simulink model "nn_plus"  (R2018b)
settings: Solver=VariableStepAuto  StartTime=0.0  StopTime=10.0  RelTol=1e-3
libraries: neural x265
(part 2 of 2)

== system nn_plus/LSTM SHA2/LSTMM Cell (with XOR|AND|SUM encapsulation)1/LSTM | XOR |AND (NN)/SUM NN/LSTM Cell [t] ==
  C[t-1] : Inport
  h[t-1] : Inport  Port=2
  X1 : Inport  Port=3
  X2 : Inport  Port=4
  Product : Product
  Product1 : Product
  Sum : Sum  Inputs=|++
  Sum1 : Sum  Inputs=|++
  Vector Concatenate : Concatenate  NumInputs=3
  logsig : neural/Transfer Functions/logsig
  logsig1 : neural/Transfer Functions/logsig
  logsig2 : neural/Transfer Functions/logsig
  tansig3 : neural/Transfer Functions/tansig
  tansig4 : neural/Transfer Functions/tansig
  C[t] : Outport
  h[t] : Outport  Port=2
  wires:
  h[t-1]/1 -> Vector Concatenate/1
  X1/1 -> Vector Concatenate/2
  X2/1 -> Vector Concatenate/3
  Vector Concatenate/1 -> tansig3/1, logsig2/1, logsig1/1, logsig/1
  C[t-1]/1 -> Sum/1
  logsig/1 -> Sum/2
  Sum/1 -> Sum1/1
  tansig3/1 -> Product/2
  logsig1/1 -> Product/1
  Product/1 -> Sum1/2
  logsig2/1 -> Product1/2
  Sum1/1 -> C[t]/1, tansig4/1
  tansig4/1 -> Product1/1
  Product1/1 -> h[t]/1

== system nn_plus/LSTM SHA2/LSTMM Cell (with XOR|AND|SUM encapsulation)1/LSTM | XOR |AND (NN)/SUM NN/LSTM Cell[t=1] ==
  note: LSTM Cell L1 (Block-Scheme)
  C[t-1] : Inport
  h[t-1] : Inport  Port=2
  X1 : Inport  Port=3
  X2 : Inport  Port=4
  Product : Product
  Product1 : Product
  Sum : Sum  Inputs=|++
  Sum1 : Sum  Inputs=|++
  Vector Concatenate : Concatenate  NumInputs=3
  logsig : neural/Transfer Functions/logsig
  logsig1 : neural/Transfer Functions/logsig
  logsig2 : neural/Transfer Functions/logsig
  tansig3 : neural/Transfer Functions/tansig
  tansig4 : neural/Transfer Functions/tansig
  C[t] : Outport
  h[t] : Outport  Port=2
  wires:
  h[t-1]/1 -> Vector Concatenate/1
  X1/1 -> Vector Concatenate/2
  X2/1 -> Vector Concatenate/3
  Vector Concatenate/1 -> logsig/1, logsig2/1, tansig3/1, logsig1/1
  C[t-1]/1 -> Sum/1
  logsig/1 -> Sum/2
  Sum/1 -> Sum1/1
  tansig3/1 -> Product/2
  logsig1/1 -> Product/1
  Product/1 -> Sum1/2
  logsig2/1 -> Product1/2
  Sum1/1 -> C[t]/1, tansig4/1
  tansig4/1 -> Product1/1
  Product1/1 -> h[t]/1

== system nn_plus/LSTM SHA2/LSTMM Cell (with XOR|AND|SUM encapsulation)1/LSTM | XOR |AND (NN)/SUM NN/LSTM Cell[t=2] ==
  C[t-1] : Inport
  h[t-1] : Inport  Port=2
  X1 : Inport  Port=3
  X2 : Inport  Port=4
  Product : Product
  Product1 : Product
  Sum : Sum  Inputs=|++
  Sum1 : Sum  Inputs=|++
  Vector Concatenate : Concatenate  NumInputs=3
  logsig : neural/Transfer Functions/logsig
  logsig1 : neural/Transfer Functions/logsig
  logsig2 : neural/Transfer Functions/logsig
  tansig3 : neural/Transfer Functions/tansig
  tansig4 : neural/Transfer Functions/tansig
  C[t] : Outport
  h[t] : Outport  Port=2
  wires:
  h[t-1]/1 -> Vector Concatenate/1
  X1/1 -> Vector Concatenate/2
  X2/1 -> Vector Concatenate/3
  Vector Concatenate/1 -> tansig3/1, logsig2/1, logsig1/1, logsig/1
  C[t-1]/1 -> Sum/1
  logsig/1 -> Sum/2
  Sum/1 -> Sum1/1
  tansig3/1 -> Product/2
  logsig1/1 -> Product/1
  Product/1 -> Sum1/2
  logsig2/1 -> Product1/2
  Sum1/1 -> C[t]/1, tansig4/1
  tansig4/1 -> Product1/1
  Product1/1 -> h[t]/1

== system nn_plus/LSTM SHA2/LSTMM Cell (with XOR|AND|SUM encapsulation)2/LSTM | XOR |AND (NN)/SUM NN/LSTM Cell [t=31] ==
  C[t-1] : Inport
  h[t-1] : Inport  Port=2
  X1 : Inport  Port=3
  X2 : Inport  Port=4
  Product : Product
  Product1 : Product
  Sum : Sum  Inputs=|++
  Sum1 : Sum  Inputs=|++
  Vector Concatenate : Concatenate  NumInputs=3
  logsig : neural/Transfer Functions/logsig
  logsig1 : neural/Transfer Functions/logsig
  logsig2 : neural/Transfer Functions/logsig
  tansig3 : neural/Transfer Functions/tansig
  tansig4 : neural/Transfer Functions/tansig
  C[t] : Outport
  h[t] : Outport  Port=2
  wires:
  h[t-1]/1 -> Vector Concatenate/1
  X1/1 -> Vector Concatenate/2
  X2/1 -> Vector Concatenate/3
  Vector Concatenate/1 -> tansig3/1, logsig2/1, logsig1/1, logsig/1
  C[t-1]/1 -> Sum/1
  logsig/1 -> Sum/2
  Sum/1 -> Sum1/1
  tansig3/1 -> Product/2
  logsig1/1 -> Product/1
  Product/1 -> Sum1/2
  logsig2/1 -> Product1/2
  Sum1/1 -> C[t]/1, tansig4/1
  tansig4/1 -> Product1/1
  Product1/1 -> h[t]/1

== system nn_plus/LSTM SHA2/LSTMM Cell (with XOR|AND|SUM encapsulation)2/LSTM | XOR |AND (NN)/SUM NN/LSTM Cell [t] ==
  C[t-1] : Inport
  h[t-1] : Inport  Port=2
  X1 : Inport  Port=3
  X2 : Inport  Port=4
  Product : Product
  Product1 : Product
  Sum : Sum  Inputs=|++
  Sum1 : Sum  Inputs=|++
  Vector Concatenate : Concatenate  NumInputs=3
  logsig : neural/Transfer Functions/logsig
  logsig1 : neural/Transfer Functions/logsig
  logsig2 : neural/Transfer Functions/logsig
  tansig3 : neural/Transfer Functions/tansig
  tansig4 : neural/Transfer Functions/tansig
  C[t] : Outport
  h[t] : Outport  Port=2
  wires:
  h[t-1]/1 -> Vector Concatenate/1
  X1/1 -> Vector Concatenate/2
  X2/1 -> Vector Concatenate/3
  Vector Concatenate/1 -> tansig3/1, logsig2/1, logsig1/1, logsig/1
  C[t-1]/1 -> Sum/1
  logsig/1 -> Sum/2
  Sum/1 -> Sum1/1
  tansig3/1 -> Product/2
  logsig1/1 -> Product/1
  Product/1 -> Sum1/2
  logsig2/1 -> Product1/2
  Sum1/1 -> C[t]/1, tansig4/1
  tansig4/1 -> Product1/1
  Product1/1 -> h[t]/1

== system nn_plus/LSTM SHA2/LSTMM Cell (with XOR|AND|SUM encapsulation)2/LSTM | XOR |AND (NN)/SUM NN/LSTM Cell[t=1] ==
  note: LSTM Cell L1 (Block-Scheme)
  C[t-1] : Inport
  h[t-1] : Inport  Port=2
  X1 : Inport  Port=3
  X2 : Inport  Port=4
  Product : Product
  Product1 : Product
  Sum : Sum  Inputs=|++
  Sum1 : Sum  Inputs=|++
  Vector Concatenate : Concatenate  NumInputs=3
  logsig : neural/Transfer Functions/logsig
  logsig1 : neural/Transfer Functions/logsig
  logsig2 : neural/Transfer Functions/logsig
  tansig3 : neural/Transfer Functions/tansig
  tansig4 : neural/Transfer Functions/tansig
  C[t] : Outport
  h[t] : Outport  Port=2
  wires:
  h[t-1]/1 -> Vector Concatenate/1
  X1/1 -> Vector Concatenate/2
  X2/1 -> Vector Concatenate/3
  Vector Concatenate/1 -> logsig/1, logsig2/1, tansig3/1, logsig1/1
  C[t-1]/1 -> Sum/1
  logsig/1 -> Sum/2
  Sum/1 -> Sum1/1
  tansig3/1 -> Product/2
  logsig1/1 -> Product/1
  Product/1 -> Sum1/2
  logsig2/1 -> Product1/2
  Sum1/1 -> C[t]/1, tansig4/1
  tansig4/1 -> Product1/1
  Product1/1 -> h[t]/1

== system nn_plus/LSTM SHA2/LSTMM Cell (with XOR|AND|SUM encapsulation)2/LSTM | XOR |AND (NN)/SUM NN/LSTM Cell[t=2] ==
  C[t-1] : Inport
  h[t-1] : Inport  Port=2
  X1 : Inport  Port=3
  X2 : Inport  Port=4
  Product : Product
  Product1 : Product
  Sum : Sum  Inputs=|++
  Sum1 : Sum  Inputs=|++
  Vector Concatenate : Concatenate  NumInputs=3
  logsig : neural/Transfer Functions/logsig
  logsig1 : neural/Transfer Functions/logsig
  logsig2 : neural/Transfer Functions/logsig
  tansig3 : neural/Transfer Functions/tansig
  tansig4 : neural/Transfer Functions/tansig
  C[t] : Outport
  h[t] : Outport  Port=2
  wires:
  h[t-1]/1 -> Vector Concatenate/1
  X1/1 -> Vector Concatenate/2
  X2/1 -> Vector Concatenate/3
  Vector Concatenate/1 -> tansig3/1, logsig2/1, logsig1/1, logsig/1
  C[t-1]/1 -> Sum/1
  logsig/1 -> Sum/2
  Sum/1 -> Sum1/1
  tansig3/1 -> Product/2
  logsig1/1 -> Product/1
  Product/1 -> Sum1/2
  logsig2/1 -> Product1/2
  Sum1/1 -> C[t]/1, tansig4/1
  tansig4/1 -> Product1/1
  Product1/1 -> h[t]/1

== system nn_plus/LSTM SHA2/LSTMM Cell (with XOR|AND|SUM encapsulation)3/LSTM | XOR |AND (NN)/SUM NN/LSTM Cell [t=31] ==
  C[t-1] : Inport
  h[t-1] : Inport  Port=2
  X1 : Inport  Port=3
  X2 : Inport  Port=4
  Product : Product
  Product1 : Product
  Sum : Sum  Inputs=|++
  Sum1 : Sum  Inputs=|++
  Vector Concatenate : Concatenate  NumInputs=3
  logsig : neural/Transfer Functions/logsig
  logsig1 : neural/Transfer Functions/logsig
  logsig2 : neural/Transfer Functions/logsig
  tansig3 : neural/Transfer Functions/tansig
  tansig4 : neural/Transfer Functions/tansig
  C[t] : Outport
  h[t] : Outport  Port=2
  wires:
  h[t-1]/1 -> Vector Concatenate/1
  X1/1 -> Vector Concatenate/2
  X2/1 -> Vector Concatenate/3
  Vector Concatenate/1 -> tansig3/1, logsig2/1, logsig1/1, logsig/1
  C[t-1]/1 -> Sum/1
  logsig/1 -> Sum/2
  Sum/1 -> Sum1/1
  tansig3/1 -> Product/2
  logsig1/1 -> Product/1
  Product/1 -> Sum1/2
  logsig2/1 -> Product1/2
  Sum1/1 -> C[t]/1, tansig4/1
  tansig4/1 -> Product1/1
  Product1/1 -> h[t]/1

== system nn_plus/LSTM SHA2/LSTMM Cell (with XOR|AND|SUM encapsulation)3/LSTM | XOR |AND (NN)/SUM NN/LSTM Cell [t] ==
  C[t-1] : Inport
  h[t-1] : Inport  Port=2
  X1 : Inport  Port=3
  X2 : Inport  Port=4
  Product : Product
  Product1 : Product
  Sum : Sum  Inputs=|++
  Sum1 : Sum  Inputs=|++
  Vector Concatenate : Concatenate  NumInputs=3
  logsig : neural/Transfer Functions/logsig
  logsig1 : neural/Transfer Functions/logsig
  logsig2 : neural/Transfer Functions/logsig
  tansig3 : neural/Transfer Functions/tansig
  tansig4 : neural/Transfer Functions/tansig
  C[t] : Outport
  h[t] : Outport  Port=2
  wires:
  h[t-1]/1 -> Vector Concatenate/1
  X1/1 -> Vector Concatenate/2
  X2/1 -> Vector Concatenate/3
  Vector Concatenate/1 -> tansig3/1, logsig2/1, logsig1/1, logsig/1
  C[t-1]/1 -> Sum/1
  logsig/1 -> Sum/2
  Sum/1 -> Sum1/1
  tansig3/1 -> Product/2
  logsig1/1 -> Product/1
  Product/1 -> Sum1/2
  logsig2/1 -> Product1/2
  Sum1/1 -> C[t]/1, tansig4/1
  tansig4/1 -> Product1/1
  Product1/1 -> h[t]/1

== system nn_plus/LSTM SHA2/LSTMM Cell (with XOR|AND|SUM encapsulation)3/LSTM | XOR |AND (NN)/SUM NN/LSTM Cell[t=1] ==
  note: LSTM Cell L1 (Block-Scheme)
  C[t-1] : Inport
  h[t-1] : Inport  Port=2
  X1 : Inport  Port=3
  X2 : Inport  Port=4
  Product : Product
  Product1 : Product
  Sum : Sum  Inputs=|++
  Sum1 : Sum  Inputs=|++
  Vector Concatenate : Concatenate  NumInputs=3
  logsig : neural/Transfer Functions/logsig
  logsig1 : neural/Transfer Functions/logsig
  logsig2 : neural/Transfer Functions/logsig
  tansig3 : neural/Transfer Functions/tansig
  tansig4 : neural/Transfer Functions/tansig
  C[t] : Outport
  h[t] : Outport  Port=2
  wires:
  h[t-1]/1 -> Vector Concatenate/1
  X1/1 -> Vector Concatenate/2
  X2/1 -> Vector Concatenate/3
  Vector Concatenate/1 -> logsig/1, logsig2/1, tansig3/1, logsig1/1
  C[t-1]/1 -> Sum/1
  logsig/1 -> Sum/2
  Sum/1 -> Sum1/1
  tansig3/1 -> Product/2
  logsig1/1 -> Product/1
  Product/1 -> Sum1/2
  logsig2/1 -> Product1/2
  Sum1/1 -> C[t]/1, tansig4/1
  tansig4/1 -> Product1/1
  Product1/1 -> h[t]/1

== system nn_plus/LSTM SHA2/LSTMM Cell (with XOR|AND|SUM encapsulation)3/LSTM | XOR |AND (NN)/SUM NN/LSTM Cell[t=2] ==
  C[t-1] : Inport
  h[t-1] : Inport  Port=2
  X1 : Inport  Port=3
  X2 : Inport  Port=4
  Product : Product
  Product1 : Product
  Sum : Sum  Inputs=|++
  Sum1 : Sum  Inputs=|++
  Vector Concatenate : Concatenate  NumInputs=3
  logsig : neural/Transfer Functions/logsig
  logsig1 : neural/Transfer Functions/logsig
  logsig2 : neural/Transfer Functions/logsig
  tansig3 : neural/Transfer Functions/tansig
  tansig4 : neural/Transfer Functions/tansig
  C[t] : Outport
  h[t] : Outport  Port=2
  wires:
  h[t-1]/1 -> Vector Concatenate/1
  X1/1 -> Vector Concatenate/2
  X2/1 -> Vector Concatenate/3
  Vector Concatenate/1 -> tansig3/1, logsig2/1, logsig1/1, logsig/1
  C[t-1]/1 -> Sum/1
  logsig/1 -> Sum/2
  Sum/1 -> Sum1/1
  tansig3/1 -> Product/2
  logsig1/1 -> Product/1
  Product/1 -> Sum1/2
  logsig2/1 -> Product1/2
  Sum1/1 -> C[t]/1, tansig4/1
  tansig4/1 -> Product1/1
  Product1/1 -> h[t]/1

== system nn_plus/LSTM SHA2/LSTMM Cell (with XOR|AND|SUM encapsulation)4/LSTM | XOR |AND (NN)/SUM NN/LSTM Cell [t=31] ==
  C[t-1] : Inport
  h[t-1] : Inport  Port=2
  X1 : Inport  Port=3
  X2 : Inport  Port=4
  Product : Product
  Product1 : Product
  Sum : Sum  Inputs=|++
  Sum1 : Sum  Inputs=|++
  Vector Concatenate : Concatenate  NumInputs=3
  logsig : neural/Transfer Functions/logsig
  logsig1 : neural/Transfer Functions/logsig
  logsig2 : neural/Transfer Functions/logsig
  tansig3 : neural/Transfer Functions/tansig
  tansig4 : neural/Transfer Functions/tansig
  C[t] : Outport
  h[t] : Outport  Port=2
  wires:
  h[t-1]/1 -> Vector Concatenate/1
  X1/1 -> Vector Concatenate/2
  X2/1 -> Vector Concatenate/3
  Vector Concatenate/1 -> tansig3/1, logsig2/1, logsig1/1, logsig/1
  C[t-1]/1 -> Sum/1
  logsig/1 -> Sum/2
  Sum/1 -> Sum1/1
  tansig3/1 -> Product/2
  logsig1/1 -> Product/1
  Product/1 -> Sum1/2
  logsig2/1 -> Product1/2
  Sum1/1 -> C[t]/1, tansig4/1
  tansig4/1 -> Product1/1
  Product1/1 -> h[t]/1

== system nn_plus/LSTM SHA2/LSTMM Cell (with XOR|AND|SUM encapsulation)4/LSTM | XOR |AND (NN)/SUM NN/LSTM Cell [t] ==
  C[t-1] : Inport
  h[t-1] : Inport  Port=2
  X1 : Inport  Port=3
  X2 : Inport  Port=4
  Product : Product
  Product1 : Product
  Sum : Sum  Inputs=|++
  Sum1 : Sum  Inputs=|++
  Vector Concatenate : Concatenate  NumInputs=3
  logsig : neural/Transfer Functions/logsig
  logsig1 : neural/Transfer Functions/logsig
  logsig2 : neural/Transfer Functions/logsig
  tansig3 : neural/Transfer Functions/tansig
  tansig4 : neural/Transfer Functions/tansig
  C[t] : Outport
  h[t] : Outport  Port=2
  wires:
  h[t-1]/1 -> Vector Concatenate/1
  X1/1 -> Vector Concatenate/2
  X2/1 -> Vector Concatenate/3
  Vector Concatenate/1 -> tansig3/1, logsig2/1, logsig1/1, logsig/1
  C[t-1]/1 -> Sum/1
  logsig/1 -> Sum/2
  Sum/1 -> Sum1/1
  tansig3/1 -> Product/2
  logsig1/1 -> Product/1
  Product/1 -> Sum1/2
  logsig2/1 -> Product1/2
  Sum1/1 -> C[t]/1, tansig4/1
  tansig4/1 -> Product1/1
  Product1/1 -> h[t]/1

== system nn_plus/LSTM SHA2/LSTMM Cell (with XOR|AND|SUM encapsulation)4/LSTM | XOR |AND (NN)/SUM NN/LSTM Cell[t=1] ==
  note: LSTM Cell L1 (Block-Scheme)
  C[t-1] : Inport
  h[t-1] : Inport  Port=2
  X1 : Inport  Port=3
  X2 : Inport  Port=4
  Product : Product
  Product1 : Product
  Sum : Sum  Inputs=|++
  Sum1 : Sum  Inputs=|++
  Vector Concatenate : Concatenate  NumInputs=3
  logsig : neural/Transfer Functions/logsig
  logsig1 : neural/Transfer Functions/logsig
  logsig2 : neural/Transfer Functions/logsig
  tansig3 : neural/Transfer Functions/tansig
  tansig4 : neural/Transfer Functions/tansig
  C[t] : Outport
  h[t] : Outport  Port=2
  wires:
  h[t-1]/1 -> Vector Concatenate/1
  X1/1 -> Vector Concatenate/2
  X2/1 -> Vector Concatenate/3
  Vector Concatenate/1 -> logsig/1, logsig2/1, tansig3/1, logsig1/1
  C[t-1]/1 -> Sum/1
  logsig/1 -> Sum/2
  Sum/1 -> Sum1/1
  tansig3/1 -> Product/2
  logsig1/1 -> Product/1
  Product/1 -> Sum1/2
  logsig2/1 -> Product1/2
  Sum1/1 -> C[t]/1, tansig4/1
  tansig4/1 -> Product1/1
  Product1/1 -> h[t]/1

== system nn_plus/LSTM SHA2/LSTMM Cell (with XOR|AND|SUM encapsulation)4/LSTM | XOR |AND (NN)/SUM NN/LSTM Cell[t=2] ==
  C[t-1] : Inport
  h[t-1] : Inport  Port=2
  X1 : Inport  Port=3
  X2 : Inport  Port=4
  Product : Product
  Product1 : Product
  Sum : Sum  Inputs=|++
  Sum1 : Sum  Inputs=|++
  Vector Concatenate : Concatenate  NumInputs=3
  logsig : neural/Transfer Functions/logsig
  logsig1 : neural/Transfer Functions/logsig
  logsig2 : neural/Transfer Functions/logsig
  tansig3 : neural/Transfer Functions/tansig
  tansig4 : neural/Transfer Functions/tansig
  C[t] : Outport
  h[t] : Outport  Port=2
  wires:
  h[t-1]/1 -> Vector Concatenate/1
  X1/1 -> Vector Concatenate/2
  X2/1 -> Vector Concatenate/3
  Vector Concatenate/1 -> tansig3/1, logsig2/1, logsig1/1, logsig/1
  C[t-1]/1 -> Sum/1
  logsig/1 -> Sum/2
  Sum/1 -> Sum1/1
  tansig3/1 -> Product/2
  logsig1/1 -> Product/1
  Product/1 -> Sum1/2
  logsig2/1 -> Product1/2
  Sum1/1 -> C[t]/1, tansig4/1
  tansig4/1 -> Product1/1
  Product1/1 -> h[t]/1

== system nn_plus/LSTM SHA2/LSTMM Cell (with XOR|AND|SUM encapsulation)5/LSTM | XOR |AND (NN)/SUM NN/LSTM Cell [t=31] ==
  C[t-1] : Inport
  h[t-1] : Inport  Port=2
  X1 : Inport  Port=3
  X2 : Inport  Port=4
  Product : Product
  Product1 : Product
  Sum : Sum  Inputs=|++
  Sum1 : Sum  Inputs=|++
  Vector Concatenate : Concatenate  NumInputs=3
  logsig : neural/Transfer Functions/logsig
  logsig1 : neural/Transfer Functions/logsig
  logsig2 : neural/Transfer Functions/logsig
  tansig3 : neural/Transfer Functions/tansig
  tansig4 : neural/Transfer Functions/tansig
  C[t] : Outport
  h[t] : Outport  Port=2
  wires:
  h[t-1]/1 -> Vector Concatenate/1
  X1/1 -> Vector Concatenate/2
  X2/1 -> Vector Concatenate/3
  Vector Concatenate/1 -> tansig3/1, logsig2/1, logsig1/1, logsig/1
  C[t-1]/1 -> Sum/1
  logsig/1 -> Sum/2
  Sum/1 -> Sum1/1
  tansig3/1 -> Product/2
  logsig1/1 -> Product/1
  Product/1 -> Sum1/2
  logsig2/1 -> Product1/2
  Sum1/1 -> C[t]/1, tansig4/1
  tansig4/1 -> Product1/1
  Product1/1 -> h[t]/1

== system nn_plus/LSTM SHA2/LSTMM Cell (with XOR|AND|SUM encapsulation)5/LSTM | XOR |AND (NN)/SUM NN/LSTM Cell [t] ==
  C[t-1] : Inport
  h[t-1] : Inport  Port=2
  X1 : Inport  Port=3
  X2 : Inport  Port=4
  Product : Product
  Product1 : Product
  Sum : Sum  Inputs=|++
  Sum1 : Sum  Inputs=|++
  Vector Concatenate : Concatenate  NumInputs=3
  logsig : neural/Transfer Functions/logsig
  logsig1 : neural/Transfer Functions/logsig
  logsig2 : neural/Transfer Functions/logsig
  tansig3 : neural/Transfer Functions/tansig
  tansig4 : neural/Transfer Functions/tansig
  C[t] : Outport
  h[t] : Outport  Port=2
  wires:
  h[t-1]/1 -> Vector Concatenate/1
  X1/1 -> Vector Concatenate/2
  X2/1 -> Vector Concatenate/3
  Vector Concatenate/1 -> tansig3/1, logsig2/1, logsig1/1, logsig/1
  C[t-1]/1 -> Sum/1
  logsig/1 -> Sum/2
  Sum/1 -> Sum1/1
  tansig3/1 -> Product/2
  logsig1/1 -> Product/1
  Product/1 -> Sum1/2
  logsig2/1 -> Product1/2
  Sum1/1 -> C[t]/1, tansig4/1
  tansig4/1 -> Product1/1
  Product1/1 -> h[t]/1

== system nn_plus/LSTM SHA2/LSTMM Cell (with XOR|AND|SUM encapsulation)5/LSTM | XOR |AND (NN)/SUM NN/LSTM Cell[t=1] ==
  note: LSTM Cell L1 (Block-Scheme)
  C[t-1] : Inport
  h[t-1] : Inport  Port=2
  X1 : Inport  Port=3
  X2 : Inport  Port=4
  Product : Product
  Product1 : Product
  Sum : Sum  Inputs=|++
  Sum1 : Sum  Inputs=|++
  Vector Concatenate : Concatenate  NumInputs=3
  logsig : neural/Transfer Functions/logsig
  logsig1 : neural/Transfer Functions/logsig
  logsig2 : neural/Transfer Functions/logsig
  tansig3 : neural/Transfer Functions/tansig
  tansig4 : neural/Transfer Functions/tansig
  C[t] : Outport
  h[t] : Outport  Port=2
  wires:
  h[t-1]/1 -> Vector Concatenate/1
  X1/1 -> Vector Concatenate/2
  X2/1 -> Vector Concatenate/3
  Vector Concatenate/1 -> logsig/1, logsig2/1, tansig3/1, logsig1/1
  C[t-1]/1 -> Sum/1
  logsig/1 -> Sum/2
  Sum/1 -> Sum1/1
  tansig3/1 -> Product/2
  logsig1/1 -> Product/1
  Product/1 -> Sum1/2
  logsig2/1 -> Product1/2
  Sum1/1 -> C[t]/1, tansig4/1
  tansig4/1 -> Product1/1
  Product1/1 -> h[t]/1

== system nn_plus/LSTM SHA2/LSTMM Cell (with XOR|AND|SUM encapsulation)5/LSTM | XOR |AND (NN)/SUM NN/LSTM Cell[t=2] ==
  C[t-1] : Inport
  h[t-1] : Inport  Port=2
  X1 : Inport  Port=3
  X2 : Inport  Port=4
  Product : Product
  Product1 : Product
  Sum : Sum  Inputs=|++
  Sum1 : Sum  Inputs=|++
  Vector Concatenate : Concatenate  NumInputs=3
  logsig : neural/Transfer Functions/logsig
  logsig1 : neural/Transfer Functions/logsig
  logsig2 : neural/Transfer Functions/logsig
  tansig3 : neural/Transfer Functions/tansig
  tansig4 : neural/Transfer Functions/tansig
  C[t] : Outport
  h[t] : Outport  Port=2
  wires:
  h[t-1]/1 -> Vector Concatenate/1
  X1/1 -> Vector Concatenate/2
  X2/1 -> Vector Concatenate/3
  Vector Concatenate/1 -> tansig3/1, logsig2/1, logsig1/1, logsig/1
  C[t-1]/1 -> Sum/1
  logsig/1 -> Sum/2
  Sum/1 -> Sum1/1
  tansig3/1 -> Product/2
  logsig1/1 -> Product/1
  Product/1 -> Sum1/2
  logsig2/1 -> Product1/2
  Sum1/1 -> C[t]/1, tansig4/1
  tansig4/1 -> Product1/1
  Product1/1 -> h[t]/1

== system nn_plus/LSTM SHA2/LSTMM Cell (with XOR|AND|SUM encapsulation)6/LSTM | XOR |AND (NN)/SUM NN/LSTM Cell [t=31] ==
  C[t-1] : Inport
  h[t-1] : Inport  Port=2
  X1 : Inport  Port=3
  X2 : Inport  Port=4
  Product : Product
  Product1 : Product
  Sum : Sum  Inputs=|++
  Sum1 : Sum  Inputs=|++
  Vector Concatenate : Concatenate  NumInputs=3
  logsig : neural/Transfer Functions/logsig
  logsig1 : neural/Transfer Functions/logsig
  logsig2 : neural/Transfer Functions/logsig
  tansig3 : neural/Transfer Functions/tansig
  tansig4 : neural/Transfer Functions/tansig
  C[t] : Outport
  h[t] : Outport  Port=2
  wires:
  h[t-1]/1 -> Vector Concatenate/1
  X1/1 -> Vector Concatenate/2
  X2/1 -> Vector Concatenate/3
  Vector Concatenate/1 -> tansig3/1, logsig2/1, logsig1/1, logsig/1
  C[t-1]/1 -> Sum/1
  logsig/1 -> Sum/2
  Sum/1 -> Sum1/1
  tansig3/1 -> Product/2
  logsig1/1 -> Product/1
  Product/1 -> Sum1/2
  logsig2/1 -> Product1/2
  Sum1/1 -> C[t]/1, tansig4/1
  tansig4/1 -> Product1/1
  Product1/1 -> h[t]/1

== system nn_plus/LSTM SHA2/LSTMM Cell (with XOR|AND|SUM encapsulation)6/LSTM | XOR |AND (NN)/SUM NN/LSTM Cell [t] ==
  C[t-1] : Inport
  h[t-1] : Inport  Port=2
  X1 : Inport  Port=3
  X2 : Inport  Port=4
  Product : Product
  Product1 : Product
  Sum : Sum  Inputs=|++
  Sum1 : Sum  Inputs=|++
  Vector Concatenate : Concatenate  NumInputs=3
  logsig : neural/Transfer Functions/logsig
  logsig1 : neural/Transfer Functions/logsig
  logsig2 : neural/Transfer Functions/logsig
  tansig3 : neural/Transfer Functions/tansig
  tansig4 : neural/Transfer Functions/tansig
  C[t] : Outport
  h[t] : Outport  Port=2
  wires:
  h[t-1]/1 -> Vector Concatenate/1
  X1/1 -> Vector Concatenate/2
  X2/1 -> Vector Concatenate/3
  Vector Concatenate/1 -> tansig3/1, logsig2/1, logsig1/1, logsig/1
  C[t-1]/1 -> Sum/1
  logsig/1 -> Sum/2
  Sum/1 -> Sum1/1
  tansig3/1 -> Product/2
  logsig1/1 -> Product/1
  Product/1 -> Sum1/2
  logsig2/1 -> Product1/2
  Sum1/1 -> C[t]/1, tansig4/1
  tansig4/1 -> Product1/1
  Product1/1 -> h[t]/1

== system nn_plus/LSTM SHA2/LSTMM Cell (with XOR|AND|SUM encapsulation)6/LSTM | XOR |AND (NN)/SUM NN/LSTM Cell[t=1] ==
  note: LSTM Cell L1 (Block-Scheme)
  C[t-1] : Inport
  h[t-1] : Inport  Port=2
  X1 : Inport  Port=3
  X2 : Inport  Port=4
  Product : Product
  Product1 : Product
  Sum : Sum  Inputs=|++
  Sum1 : Sum  Inputs=|++
  Vector Concatenate : Concatenate  NumInputs=3
  logsig : neural/Transfer Functions/logsig
  logsig1 : neural/Transfer Functions/logsig
  logsig2 : neural/Transfer Functions/logsig
  tansig3 : neural/Transfer Functions/tansig
  tansig4 : neural/Transfer Functions/tansig
  C[t] : Outport
  h[t] : Outport  Port=2
  wires:
  h[t-1]/1 -> Vector Concatenate/1
  X1/1 -> Vector Concatenate/2
  X2/1 -> Vector Concatenate/3
  Vector Concatenate/1 -> logsig/1, logsig2/1, tansig3/1, logsig1/1
  C[t-1]/1 -> Sum/1
  logsig/1 -> Sum/2
  Sum/1 -> Sum1/1
  tansig3/1 -> Product/2
  logsig1/1 -> Product/1
  Product/1 -> Sum1/2
  logsig2/1 -> Product1/2
  Sum1/1 -> C[t]/1, tansig4/1
  tansig4/1 -> Product1/1
  Product1/1 -> h[t]/1

== system nn_plus/LSTM SHA2/LSTMM Cell (with XOR|AND|SUM encapsulation)6/LSTM | XOR |AND (NN)/SUM NN/LSTM Cell[t=2] ==
  C[t-1] : Inport
  h[t-1] : Inport  Port=2
  X1 : Inport  Port=3
  X2 : Inport  Port=4
  Product : Product
  Product1 : Product
  Sum : Sum  Inputs=|++
  Sum1 : Sum  Inputs=|++
  Vector Concatenate : Concatenate  NumInputs=3
  logsig : neural/Transfer Functions/logsig
  logsig1 : neural/Transfer Functions/logsig
  logsig2 : neural/Transfer Functions/logsig
  tansig3 : neural/Transfer Functions/tansig
  tansig4 : neural/Transfer Functions/tansig
  C[t] : Outport
  h[t] : Outport  Port=2
  wires:
  h[t-1]/1 -> Vector Concatenate/1
  X1/1 -> Vector Concatenate/2
  X2/1 -> Vector Concatenate/3
  Vector Concatenate/1 -> tansig3/1, logsig2/1, logsig1/1, logsig/1
  C[t-1]/1 -> Sum/1
  logsig/1 -> Sum/2
  Sum/1 -> Sum1/1
  tansig3/1 -> Product/2
  logsig1/1 -> Product/1
  Product/1 -> Sum1/2
  logsig2/1 -> Product1/2
  Sum1/1 -> C[t]/1, tansig4/1
  tansig4/1 -> Product1/1
  Product1/1 -> h[t]/1

== system nn_plus/LSTM SHA2/LSTMM Cell (with XOR|AND|SUM encapsulation)7/LSTM | XOR |AND (NN)/SUM NN/LSTM Cell [t=31] ==
  C[t-1] : Inport
  h[t-1] : Inport  Port=2
  X1 : Inport  Port=3
  X2 : Inport  Port=4
  Product : Product
  Product1 : Product
  Sum : Sum  Inputs=|++
  Sum1 : Sum  Inputs=|++
  Vector Concatenate : Concatenate  NumInputs=3
  logsig : neural/Transfer Functions/logsig
  logsig1 : neural/Transfer Functions/logsig
  logsig2 : neural/Transfer Functions/logsig
  tansig3 : neural/Transfer Functions/tansig
  tansig4 : neural/Transfer Functions/tansig
  C[t] : Outport
  h[t] : Outport  Port=2
  wires:
  h[t-1]/1 -> Vector Concatenate/1
  X1/1 -> Vector Concatenate/2
  X2/1 -> Vector Concatenate/3
  Vector Concatenate/1 -> tansig3/1, logsig2/1, logsig1/1, logsig/1
  C[t-1]/1 -> Sum/1
  logsig/1 -> Sum/2
  Sum/1 -> Sum1/1
  tansig3/1 -> Product/2
  logsig1/1 -> Product/1
  Product/1 -> Sum1/2
  logsig2/1 -> Product1/2
  Sum1/1 -> C[t]/1, tansig4/1
  tansig4/1 -> Product1/1
  Product1/1 -> h[t]/1

== system nn_plus/LSTM SHA2/LSTMM Cell (with XOR|AND|SUM encapsulation)7/LSTM | XOR |AND (NN)/SUM NN/LSTM Cell [t] ==
  C[t-1] : Inport
  h[t-1] : Inport  Port=2
  X1 : Inport  Port=3
  X2 : Inport  Port=4
  Product : Product
  Product1 : Product
  Sum : Sum  Inputs=|++
  Sum1 : Sum  Inputs=|++
  Vector Concatenate : Concatenate  NumInputs=3
  logsig : neural/Transfer Functions/logsig
  logsig1 : neural/Transfer Functions/logsig
  logsig2 : neural/Transfer Functions/logsig
  tansig3 : neural/Transfer Functions/tansig
  tansig4 : neural/Transfer Functions/tansig
  C[t] : Outport
  h[t] : Outport  Port=2
  wires:
  h[t-1]/1 -> Vector Concatenate/1
  X1/1 -> Vector Concatenate/2
  X2/1 -> Vector Concatenate/3
  Vector Concatenate/1 -> tansig3/1, logsig2/1, logsig1/1, logsig/1
  C[t-1]/1 -> Sum/1
  logsig/1 -> Sum/2
  Sum/1 -> Sum1/1
  tansig3/1 -> Product/2
  logsig1/1 -> Product/1
  Product/1 -> Sum1/2
  logsig2/1 -> Product1/2
  Sum1/1 -> C[t]/1, tansig4/1
  tansig4/1 -> Product1/1
  Product1/1 -> h[t]/1

== system nn_plus/LSTM SHA2/LSTMM Cell (with XOR|AND|SUM encapsulation)7/LSTM | XOR |AND (NN)/SUM NN/LSTM Cell[t=1] ==
  note: LSTM Cell L1 (Block-Scheme)
  C[t-1] : Inport
  h[t-1] : Inport  Port=2
  X1 : Inport  Port=3
  X2 : Inport  Port=4
  Product : Product
  Product1 : Product
  Sum : Sum  Inputs=|++
  Sum1 : Sum  Inputs=|++
  Vector Concatenate : Concatenate  NumInputs=3
  logsig : neural/Transfer Functions/logsig
  logsig1 : neural/Transfer Functions/logsig
  logsig2 : neural/Transfer Functions/logsig
  tansig3 : neural/Transfer Functions/tansig
  tansig4 : neural/Transfer Functions/tansig
  C[t] : Outport
  h[t] : Outport  Port=2
  wires:
  h[t-1]/1 -> Vector Concatenate/1
  X1/1 -> Vector Concatenate/2
  X2/1 -> Vector Concatenate/3
  Vector Concatenate/1 -> logsig/1, logsig2/1, tansig3/1, logsig1/1
  C[t-1]/1 -> Sum/1
  logsig/1 -> Sum/2
  Sum/1 -> Sum1/1
  tansig3/1 -> Product/2
  logsig1/1 -> Product/1
  Product/1 -> Sum1/2
  logsig2/1 -> Product1/2
  Sum1/1 -> C[t]/1, tansig4/1
  tansig4/1 -> Product1/1
  Product1/1 -> h[t]/1

== system nn_plus/LSTM SHA2/LSTMM Cell (with XOR|AND|SUM encapsulation)7/LSTM | XOR |AND (NN)/SUM NN/LSTM Cell[t=2] ==
  C[t-1] : Inport
  h[t-1] : Inport  Port=2
  X1 : Inport  Port=3
  X2 : Inport  Port=4
  Product : Product
  Product1 : Product
  Sum : Sum  Inputs=|++
  Sum1 : Sum  Inputs=|++
  Vector Concatenate : Concatenate  NumInputs=3
  logsig : neural/Transfer Functions/logsig
  logsig1 : neural/Transfer Functions/logsig
  logsig2 : neural/Transfer Functions/logsig
  tansig3 : neural/Transfer Functions/tansig
  tansig4 : neural/Transfer Functions/tansig
  C[t] : Outport
  h[t] : Outport  Port=2
  wires:
  h[t-1]/1 -> Vector Concatenate/1
  X1/1 -> Vector Concatenate/2
  X2/1 -> Vector Concatenate/3
  Vector Concatenate/1 -> tansig3/1, logsig2/1, logsig1/1, logsig/1
  C[t-1]/1 -> Sum/1
  logsig/1 -> Sum/2
  Sum/1 -> Sum1/1
  tansig3/1 -> Product/2
  logsig1/1 -> Product/1
  Product/1 -> Sum1/2
  logsig2/1 -> Product1/2
  Sum1/1 -> C[t]/1, tansig4/1
  tansig4/1 -> Product1/1
  Product1/1 -> h[t]/1

== system nn_plus/LSTM SHA2/LSTMM Cell (with XOR|AND|SUM encapsulation)8/LSTM | XOR |AND (NN)/SUM NN/LSTM Cell [t=31] ==
  C[t-1] : Inport
  h[t-1] : Inport  Port=2
  X1 : Inport  Port=3
  X2 : Inport  Port=4
  Product : Product
  Product1 : Product
  Sum : Sum  Inputs=|++
  Sum1 : Sum  Inputs=|++
  Vector Concatenate : Concatenate  NumInputs=3
  logsig : neural/Transfer Functions/logsig
  logsig1 : neural/Transfer Functions/logsig
  logsig2 : neural/Transfer Functions/logsig
  tansig3 : neural/Transfer Functions/tansig
  tansig4 : neural/Transfer Functions/tansig
  C[t] : Outport
  h[t] : Outport  Port=2
  wires:
  h[t-1]/1 -> Vector Concatenate/1
  X1/1 -> Vector Concatenate/2
  X2/1 -> Vector Concatenate/3
  Vector Concatenate/1 -> tansig3/1, logsig2/1, logsig1/1, logsig/1
  C[t-1]/1 -> Sum/1
  logsig/1 -> Sum/2
  Sum/1 -> Sum1/1
  tansig3/1 -> Product/2
  logsig1/1 -> Product/1
  Product/1 -> Sum1/2
  logsig2/1 -> Product1/2
  Sum1/1 -> C[t]/1, tansig4/1
  tansig4/1 -> Product1/1
  Product1/1 -> h[t]/1

== system nn_plus/LSTM SHA2/LSTMM Cell (with XOR|AND|SUM encapsulation)8/LSTM | XOR |AND (NN)/SUM NN/LSTM Cell [t] ==
  C[t-1] : Inport
  h[t-1] : Inport  Port=2
  X1 : Inport  Port=3
  X2 : Inport  Port=4
  Product : Product
  Product1 : Product
  Sum : Sum  Inputs=|++
  Sum1 : Sum  Inputs=|++
  Vector Concatenate : Concatenate  NumInputs=3
  logsig : neural/Transfer Functions/logsig
  logsig1 : neural/Transfer Functions/logsig
  logsig2 : neural/Transfer Functions/logsig
  tansig3 : neural/Transfer Functions/tansig
  tansig4 : neural/Transfer Functions/tansig
  C[t] : Outport
  h[t] : Outport  Port=2
  wires:
  h[t-1]/1 -> Vector Concatenate/1
  X1/1 -> Vector Concatenate/2
  X2/1 -> Vector Concatenate/3
  Vector Concatenate/1 -> tansig3/1, logsig2/1, logsig1/1, logsig/1
  C[t-1]/1 -> Sum/1
  logsig/1 -> Sum/2
  Sum/1 -> Sum1/1
  tansig3/1 -> Product/2
  logsig1/1 -> Product/1
  Product/1 -> Sum1/2
  logsig2/1 -> Product1/2
  Sum1/1 -> C[t]/1, tansig4/1
  tansig4/1 -> Product1/1
  Product1/1 -> h[t]/1

== system nn_plus/LSTM SHA2/LSTMM Cell (with XOR|AND|SUM encapsulation)8/LSTM | XOR |AND (NN)/SUM NN/LSTM Cell[t=1] ==
  note: LSTM Cell L1 (Block-Scheme)
  C[t-1] : Inport
  h[t-1] : Inport  Port=2
  X1 : Inport  Port=3
  X2 : Inport  Port=4
  Product : Product
  Product1 : Product
  Sum : Sum  Inputs=|++
  Sum1 : Sum  Inputs=|++
  Vector Concatenate : Concatenate  NumInputs=3
  logsig : neural/Transfer Functions/logsig
  logsig1 : neural/Transfer Functions/logsig
  logsig2 : neural/Transfer Functions/logsig
  tansig3 : neural/Transfer Functions/tansig
  tansig4 : neural/Transfer Functions/tansig
  C[t] : Outport
  h[t] : Outport  Port=2
  wires:
  h[t-1]/1 -> Vector Concatenate/1
  X1/1 -> Vector Concatenate/2
  X2/1 -> Vector Concatenate/3
  Vector Concatenate/1 -> logsig/1, logsig2/1, tansig3/1, logsig1/1
  C[t-1]/1 -> Sum/1
  logsig/1 -> Sum/2
  Sum/1 -> Sum1/1
  tansig3/1 -> Product/2
  logsig1/1 -> Product/1
  Product/1 -> Sum1/2
  logsig2/1 -> Product1/2
  Sum1/1 -> C[t]/1, tansig4/1
  tansig4/1 -> Product1/1
  Product1/1 -> h[t]/1

== system nn_plus/LSTM SHA2/LSTMM Cell (with XOR|AND|SUM encapsulation)8/LSTM | XOR |AND (NN)/SUM NN/LSTM Cell[t=2] ==
  C[t-1] : Inport
  h[t-1] : Inport  Port=2
  X1 : Inport  Port=3
  X2 : Inport  Port=4
  Product : Product
  Product1 : Product
  Sum : Sum  Inputs=|++
  Sum1 : Sum  Inputs=|++
  Vector Concatenate : Concatenate  NumInputs=3
  logsig : neural/Transfer Functions/logsig
  logsig1 : neural/Transfer Functions/logsig
  logsig2 : neural/Transfer Functions/logsig
  tansig3 : neural/Transfer Functions/tansig
  tansig4 : neural/Transfer Functions/tansig
  C[t] : Outport
  h[t] : Outport  Port=2
  wires:
  h[t-1]/1 -> Vector Concatenate/1
  X1/1 -> Vector Concatenate/2
  X2/1 -> Vector Concatenate/3
  Vector Concatenate/1 -> tansig3/1, logsig2/1, logsig1/1, logsig/1
  C[t-1]/1 -> Sum/1
  logsig/1 -> Sum/2
  Sum/1 -> Sum1/1
  tansig3/1 -> Product/2
  logsig1/1 -> Product/1
  Product/1 -> Sum1/2
  logsig2/1 -> Product1/2
  Sum1/1 -> C[t]/1, tansig4/1
  tansig4/1 -> Product1/1
  Product1/1 -> h[t]/1

== system nn_plus/LSTM SHA2/LSTMM Cell (with XOR|AND|SUM encapsulation)9/LSTM | XOR |AND (NN)/SUM NN/LSTM Cell [t=31] ==
  C[t-1] : Inport
  h[t-1] : Inport  Port=2
  X1 : Inport  Port=3
  X2 : Inport  Port=4
  Product : Product
  Product1 : Product
  Sum : Sum  Inputs=|++
  Sum1 : Sum  Inputs=|++
  Vector Concatenate : Concatenate  NumInputs=3
  logsig : neural/Transfer Functions/logsig
  logsig1 : neural/Transfer Functions/logsig
  logsig2 : neural/Transfer Functions/logsig
  tansig3 : neural/Transfer Functions/tansig
  tansig4 : neural/Transfer Functions/tansig
  C[t] : Outport
  h[t] : Outport  Port=2
  wires:
  h[t-1]/1 -> Vector Concatenate/1
  X1/1 -> Vector Concatenate/2
  X2/1 -> Vector Concatenate/3
  Vector Concatenate/1 -> tansig3/1, logsig2/1, logsig1/1, logsig/1
  C[t-1]/1 -> Sum/1
  logsig/1 -> Sum/2
  Sum/1 -> Sum1/1
  tansig3/1 -> Product/2
  logsig1/1 -> Product/1
  Product/1 -> Sum1/2
  logsig2/1 -> Product1/2
  Sum1/1 -> C[t]/1, tansig4/1
  tansig4/1 -> Product1/1
  Product1/1 -> h[t]/1

== system nn_plus/LSTM SHA2/LSTMM Cell (with XOR|AND|SUM encapsulation)9/LSTM | XOR |AND (NN)/SUM NN/LSTM Cell [t] ==
  C[t-1] : Inport
  h[t-1] : Inport  Port=2
  X1 : Inport  Port=3
  X2 : Inport  Port=4
  Product : Product
  Product1 : Product
  Sum : Sum  Inputs=|++
  Sum1 : Sum  Inputs=|++
  Vector Concatenate : Concatenate  NumInputs=3
  logsig : neural/Transfer Functions/logsig
  logsig1 : neural/Transfer Functions/logsig
  logsig2 : neural/Transfer Functions/logsig
  tansig3 : neural/Transfer Functions/tansig
  tansig4 : neural/Transfer Functions/tansig
  C[t] : Outport
  h[t] : Outport  Port=2
  wires:
  h[t-1]/1 -> Vector Concatenate/1
  X1/1 -> Vector Concatenate/2
  X2/1 -> Vector Concatenate/3
  Vector Concatenate/1 -> tansig3/1, logsig2/1, logsig1/1, logsig/1
  C[t-1]/1 -> Sum/1
  logsig/1 -> Sum/2
  Sum/1 -> Sum1/1
  tansig3/1 -> Product/2
  logsig1/1 -> Product/1
  Product/1 -> Sum1/2
  logsig2/1 -> Product1/2
  Sum1/1 -> C[t]/1, tansig4/1
  tansig4/1 -> Product1/1
  Product1/1 -> h[t]/1

== system nn_plus/LSTM SHA2/LSTMM Cell (with XOR|AND|SUM encapsulation)9/LSTM | XOR |AND (NN)/SUM NN/LSTM Cell[t=1] ==
  note: LSTM Cell L1 (Block-Scheme)
  C[t-1] : Inport
  h[t-1] : Inport  Port=2
  X1 : Inport  Port=3
  X2 : Inport  Port=4
  Product : Product
  Product1 : Product
  Sum : Sum  Inputs=|++
  Sum1 : Sum  Inputs=|++
  Vector Concatenate : Concatenate  NumInputs=3
  logsig : neural/Transfer Functions/logsig
  logsig1 : neural/Transfer Functions/logsig
  logsig2 : neural/Transfer Functions/logsig
  tansig3 : neural/Transfer Functions/tansig
  tansig4 : neural/Transfer Functions/tansig
  C[t] : Outport
  h[t] : Outport  Port=2
  wires:
  h[t-1]/1 -> Vector Concatenate/1
  X1/1 -> Vector Concatenate/2
  X2/1 -> Vector Concatenate/3
  Vector Concatenate/1 -> logsig/1, logsig2/1, tansig3/1, logsig1/1
  C[t-1]/1 -> Sum/1
  logsig/1 -> Sum/2
  Sum/1 -> Sum1/1
  tansig3/1 -> Product/2
  logsig1/1 -> Product/1
  Product/1 -> Sum1/2
  logsig2/1 -> Product1/2
  Sum1/1 -> C[t]/1, tansig4/1
  tansig4/1 -> Product1/1
  Product1/1 -> h[t]/1

== system nn_plus/LSTM SHA2/LSTMM Cell (with XOR|AND|SUM encapsulation)9/LSTM | XOR |AND (NN)/SUM NN/LSTM Cell[t=2] ==
  C[t-1] : Inport
  h[t-1] : Inport  Port=2
  X1 : Inport  Port=3
  X2 : Inport  Port=4
  Product : Product
  Product1 : Product
  Sum : Sum  Inputs=|++
  Sum1 : Sum  Inputs=|++
  Vector Concatenate : Concatenate  NumInputs=3
  logsig : neural/Transfer Functions/logsig
  logsig1 : neural/Transfer Functions/logsig
  logsig2 : neural/Transfer Functions/logsig
  tansig3 : neural/Transfer Functions/tansig
  tansig4 : neural/Transfer Functions/tansig
  C[t] : Outport
  h[t] : Outport  Port=2
  wires:
  h[t-1]/1 -> Vector Concatenate/1
  X1/1 -> Vector Concatenate/2
  X2/1 -> Vector Concatenate/3
  Vector Concatenate/1 -> tansig3/1, logsig2/1, logsig1/1, logsig/1
  C[t-1]/1 -> Sum/1
  logsig/1 -> Sum/2
  Sum/1 -> Sum1/1
  tansig3/1 -> Product/2
  logsig1/1 -> Product/1
  Product/1 -> Sum1/2
  logsig2/1 -> Product1/2
  Sum1/1 -> C[t]/1, tansig4/1
  tansig4/1 -> Product1/1
  Product1/1 -> h[t]/1
